simulink library "Cassie_CommandBlock_Library_3"  (R2017b)
settings: Solver=VariableStepAuto  StartTime=0.0  StopTime=10.0  RelTol=1e-3
undefined symbols (not defined in the file): dq, isSim, q, UserParams
libraries: Cassie_CommandBlock_Library_3 x1
settings Model: Creator=81068  LastModifiedBy=81068

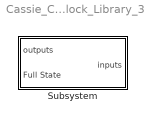
== system Cassie_CommandBlock_Library_3 ==
  Subsystem : Subsystem

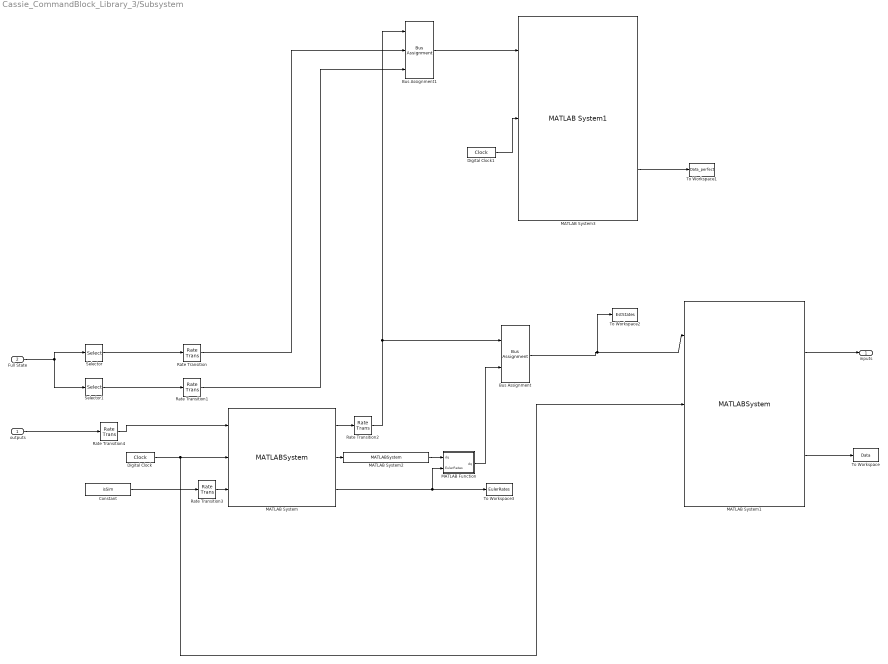
== system Cassie_CommandBlock_Library_3/Subsystem ==
  outputs : Inport  OutDataTypeStr=Bus: CassieOutBus
  Full State : Inport  Port=2
  Bus Assignment : BusAssignment  AssignedSignals=dq
  Bus Assignment1 : BusAssignment  AssignedSignals=q,dq
  Constant : Constant  Value=isSim  OutDataTypeStr=int8  LockScale=on
  Digital Clock : DigitalClock  SampleTime=UserParams.SampleTime
  Digital Clock1 : DigitalClock  SampleTime=UserParams.SampleTime
  MATLAB Function : MATLAB Function  TreatAsAtomicUnit=on
  MATLAB System : MATLABSystem  System=StateEstimator_1  step_time=0.3  SimulateUsing=Interpreted execution
      mask Type: StateEstimator_1
      mask Display:
      | disp('StateEstimator_1');
      | port_label('input',1,'cassieOutputs');
      | port_label('input',2,'t_total');
      | port_label('input',3,'isSim');
      | port_label('output',1,'EstStates');
      | port_label('output',2,'q');
      | port_label('output',3,'EulerRates');
  MATLAB System1 : MATLABSystem  System=Cassie_Controller_3  step_time=0.3  sample_time=sample_time  cov_q_measured=cov_q_measured  cov_dq_estimated=cov_dq_estimated  SimulateUsing=Code generation
      mask Type: Cassie_Controller_3
      mask Display:
      | disp('Cassie_Controller_3');
      | port_label('output',1,'userInputs');
      | port_label('output',2,'Data');
  MATLAB System2 : MATLABSystem  System=PolyRegressionFilter  sample_time=sample_time  history_length=history_length  dop=dop  signal_dim=20  delay=0  SimulateUsing=Code generation
      mask Type: PolyRegressionFilter
      mask Display:
      | disp('PolyRegressionFilter');
      | port_label('input',1,'q');
      | port_label('output',1,'dq');
  MATLAB System3 : Cassie_CommandBlock_Library_3/Subsystem/MATLAB System1  step_time=0.3  sample_time=sample_time  cov_q_measured=cov_q_measured  cov_dq_estimated=cov_dq_estimated  SimulateUsing=Code generation
  Rate Transition{,1..4} (5 alike) : RateTransition  OutPortSampleTime=sample_time
  Selector : Selector  InputPortWidth=40  IndexOptions=Index vector (dialog)  Indices=1:20  OutputSizes=1
  Selector1 : Selector  InputPortWidth=40  IndexOptions=Index vector (dialog)  Indices=21:40  OutputSizes=1
  To Workspace : ToWorkspace  VariableName=Data  SaveFormat=Timeseries  SampleTime=-1
  To Workspace1 : ToWorkspace  VariableName=Data_perfect  SaveFormat=Timeseries  SampleTime=-1
  To Workspace2 : ToWorkspace  VariableName=EstStates  SaveFormat=Timeseries  SampleTime=-1
  To Workspace3 : ToWorkspace  VariableName=EulerRates  SaveFormat=Timeseries  SampleTime=-1
  "inputs " : Outport
  wires:
  outputs/1 -> Rate Transition4/1
  MATLAB System1/2 -> To Workspace/1
  Digital Clock/1 -> MATLAB System1/2, MATLAB System/2
  Constant/1 -> Rate Transition3/1
  MATLAB System/1 -> Rate Transition2/1
  Full State/1 -> Selector1/1, Selector/1
  Selector/1 -> Rate Transition/1
  Selector1/1 -> Rate Transition1/1
  Rate Transition2/1 -> Bus Assignment/1, Bus Assignment1/1
  Rate Transition3/1 -> MATLAB System/3
  Rate Transition4/1 -> MATLAB System/1
  MATLAB System/2 -> MATLAB System2/1
  Bus Assignment1/1 -> MATLAB System3/1
  Digital Clock1/1 -> MATLAB System3/2
  Rate Transition/1 -> Bus Assignment1/2
  Rate Transition1/1 -> Bus Assignment1/3
  MATLAB System3/2 -> To Workspace1/1
  Bus Assignment/1 -> To Workspace2/1, MATLAB System1/1
  MATLAB System1/1 -> "inputs "/1
  MATLAB System/3 -> MATLAB Function/2(EulerRates), To Workspace3/1
  MATLAB System2/1 -> MATLAB Function/1("dq ")
  MATLAB Function/1(dq) -> Bus Assignment/2

== matlab function Cassie_CommandBlock_Library_3/Subsystem/MATLAB Function ==
  data: dq input; dq output; EulerRates input
function dq = mix_dq(dq,EulerRates)
dq(4:6) = EulerRates;
